simulink model "Pendulo"  (R2022b)
settings: Solver=VariableStepAuto  StartTime=0.0  StopTime=100  FixedStep=0.01  MaxStep=0.1  MinStep=0.01  RelTol=1e-3
model workspace (MAT data in the model file):
  K = 0.3
  W = 1.25
  k = 0.3
  w = 1.25
  x0 = 0
  y0 = 0
undefined symbols (not defined in the file): theta0
settings Model: NumberOfSteps=10  Creator=WINDOWS  LastModifiedBy=WINDOWS
settings DataIOCC: SaveFormat=Array  OutputTimes=tout

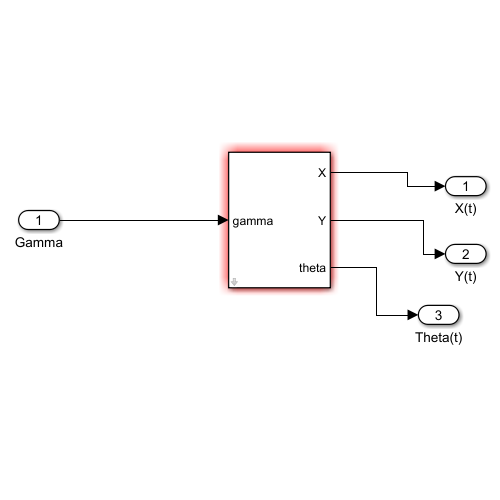
[thumbnail: Simulink's stored preview of the top-level diagram]
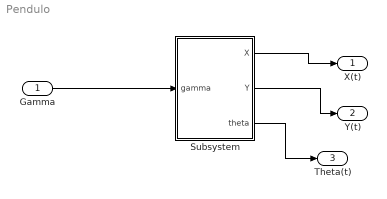
== system Pendulo ==
  Gamma : Inport
  Subsystem : Subsystem  mask{k=k, w=w, x0=x0, y0=y0, theta0=theta0}
  X(t) : Outport
  Y(t) : Outport  Port=2
  Theta(t) : Outport  Port=3
  wires:
  Subsystem/1(X) -> X(t)/1
  Subsystem/2(Y) -> Y(t)/1
  Gamma/1 -> Subsystem/1(gamma)
  Subsystem/3(theta) -> Theta(t)/1

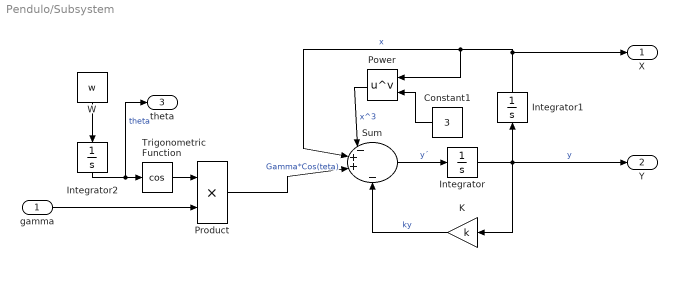
== system Pendulo/Subsystem ==
  gamma : Inport
  Constant1 : Constant  Value=3
  Integrator : Integrator  InitialCondition=y0
  Integrator1 : Integrator  InitialCondition=x0
  Integrator2 : Integrator  InitialCondition=theta0
  K : Gain  Gain=k
  Power : Math  Operator=pow
  Product : Product
  Sum : Sum  Inputs=|-++|-
  Trigonometric Function : Trigonometry  Operator=cos
  W : Constant  Value=w
  X : Outport
  Y : Outport  Port=2
  theta : Outport  Port=3
  wires:
  Trigonometric Function/1 -> Product/1
  Integrator/1 -> Y/1, K/1, Integrator1/1  "y"
  Product/1 -> Sum/3  "Gamma*Cos(teta)"
  Power/1 -> Sum/1  "x^3"
  Constant1/1 -> Power/2
  K/1 -> Sum/4  "ky"
  Integrator1/1 -> Power/1, Sum/2, X/1  "x"
  gamma/1 -> Product/2
  Sum/1 -> Integrator/1  "y´"
  Integrator2/1 -> theta/1, Trigonometric Function/1  "theta"
  W/1 -> Integrator2/1
